simulink model "my3bars"  (R2013a)
settings: Solver=ode45  StartTime=0.0  StopTime=10.0  RelTol=1e-3
values from neighbouring files (symbols this model uses):
  M1 = TwoPortBeamTxTyRz(rho,S1,l1,E,Iz1,0)    [Script_4_bars_publi_MUBO.m]
  M2 = TwoPortBeamTxTyRz(rho,S2,l2,E,Iz2,0)    [Script_4_bars_publi_MUBO.m]
  M3 = TwoPortBeamTxTyRz(rho,S3,l3,E,Iz3,0)    [Script_4_bars_publi_MUBO.m]
  mt = 0.0925*4.4482216152605/9.81    (= 0.0419429663009)    [Script_4_bars_publi_MUBO.m]
  R2 = [cos(theta2) -sin(theta2);sin(theta2) cos(theta2)]    [Script_4_bars_publi_MUBO.m]    (also in four_bars.m = zeros(3,3))
  R3 = [cos(theta3) -sin(theta3);sin(theta3) cos(theta3)]    [Script_4_bars_publi_MUBO.m]
undefined symbols (not defined in the file or in its folder): invio
libraries: cstblocks x3
settings Model: BufferReuse=off  Creator=d.alazard  LastModifiedBy=d.alazard
settings OptimizationCC: InlineParams=on  BufferReuse=off
settings DebuggingCC: InitInArrayFormatMsg=none

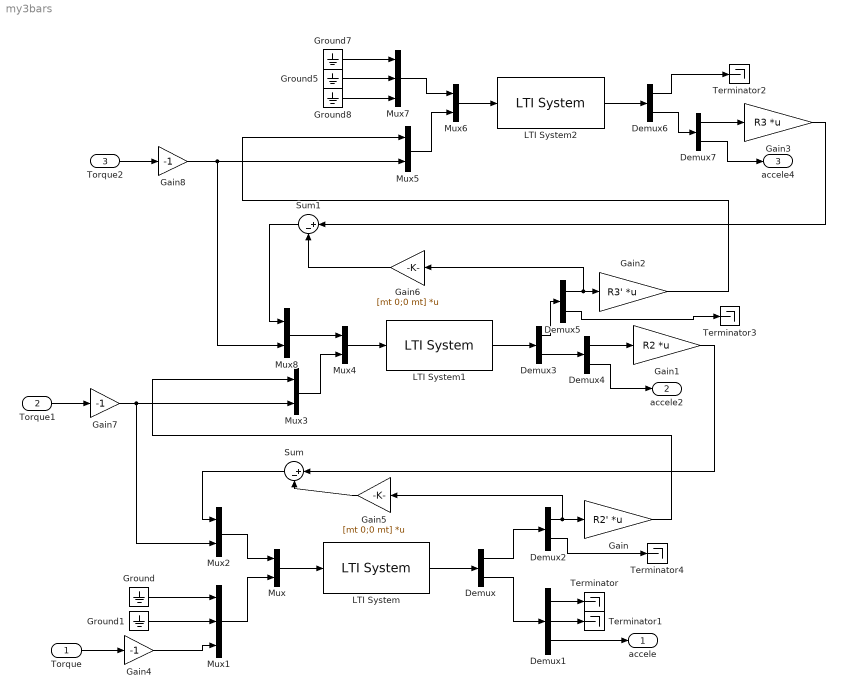
== system my3bars ==
  Torque : Inport
  Torque1 : Inport  Port=2
  Torque2 : Inport  Port=3
  Demux : Demux  Outputs=[3 3]
  Demux1 : Demux  Outputs=3
  Demux{2,4..5,7} (4 alike) : Demux  Outputs=[2 1]
  Demux3 : Demux  Outputs=[3 3]
  Demux6 : Demux  Outputs=[3 3]
  Gain : Gain  Gain=R2'  Multiplication=Matrix(K*u) (u vector)
  Gain1 : Gain  Gain=R2  Multiplication=Matrix(K*u) (u vector)
  Gain2 : Gain  Gain=R3'  Multiplication=Matrix(K*u) (u vector)
  Gain3 : Gain  Gain=R3  Multiplication=Matrix(K*u) (u vector)
  Gain4 : Gain  Gain=-1
  Gain5 : Gain  Gain=[mt 0;0 mt]  Multiplication=Matrix(K*u) (u vector)
  Gain6 : Gain  Gain=[mt 0;0 mt]  Multiplication=Matrix(K*u) (u vector)
  Gain7 : Gain  Gain=-1
  Gain8 : Gain  Gain=-1
  Ground{,1,5,7..8} (5 alike) : Ground
  LTI System : cstblocks/LTI System  sys=invio(M1,6)  IC=[]
  LTI System1 : cstblocks/LTI System  sys=invio(M2,6)  IC=[]
  LTI System2 : cstblocks/LTI System  sys=invio(M3,[1 2 6])  IC=[]
  Mux : Mux  Inputs=[3 3]
  Mux1 : Mux  Inputs=3
  Mux{2..3,5,8} (4 alike) : Mux  Inputs=[2 1]
  Mux4 : Mux  Inputs=[3 3]
  Mux6 : Mux  Inputs=[3 3]
  Mux7 : Mux  Inputs=3
  Sum : Sum  Inputs=|+-
  Sum1 : Sum  Inputs=|+-
  Terminator{,1..4} (5 alike) : Terminator
  accele : Outport
  accele2 : Outport  Port=2
  accele4 : Outport  Port=3
  wires:
  Mux/1 -> LTI System/1
  Mux1/1 -> Mux/2
  Torque/1 -> Gain4/1
  Ground/1 -> Mux1/1
  Ground1/1 -> Mux1/2
  LTI System/1 -> Demux/1
  Demux/2 -> Demux1/1
  Demux1/3 -> accele/1
  Demux1/1 -> Terminator/1
  Demux1/2 -> Terminator1/1
  Mux2/1 -> Mux/1
  Gain7/1 -> Mux2/2, Mux3/2
  Demux/1 -> Demux2/1
  Gain/1 -> Mux3/1
  Torque1/1 -> Gain7/1
  Mux3/1 -> Mux4/2
  Mux4/1 -> LTI System1/1
  LTI System1/1 -> Demux3/1
  Demux3/2 -> Demux4/1
  Demux4/1 -> Gain1/1
  Demux4/2 -> accele2/1
  Demux2/2 -> Terminator4/1
  Torque2/1 -> Gain8/1
  Mux5/1 -> Mux6/2
  Mux6/1 -> LTI System2/1
  Mux7/1 -> Mux6/1
  Ground5/1 -> Mux7/2
  Demux5/1 -> Gain6/1, Gain2/1
  Demux5/2 -> Terminator3/1
  Demux3/1 -> Demux5/1
  Gain2/1 -> Mux5/1
  Mux8/1 -> Mux4/1
  Gain8/1 -> Mux8/2, Mux5/2
  LTI System2/1 -> Demux6/1
  Demux6/2 -> Demux7/1
  Demux7/2 -> accele4/1
  Demux7/1 -> Gain3/1
  Ground7/1 -> Mux7/1
  Ground8/1 -> Mux7/3
  Demux6/1 -> Terminator2/1
  Gain4/1 -> Mux1/3
  Demux2/1 -> Gain5/1, Gain/1
  Gain5/1 -> Sum/2
  Gain1/1 -> Sum/1
  Sum/1 -> Mux2/1
  Gain6/1 -> Sum1/2
  Sum1/1 -> Mux8/1
  Gain3/1 -> Sum1/1
